simulink model "unifiedModle_IR_MAYBE"  (R2023b)
settings: Solver=FixedStepAuto  StartTime=0.0  StopTime=inf  RelTol=1e-3  EnableMultiTasking=on
libraries: vexarmcortexlib x28, vexcommonlib x8, simulink x3
settings Model: Creator=carol  LastModifiedBy=carol
settings SolverCC: AutoInsertRateTranBlk=on
settings DataIOCC: LimitDataPoints=on  SignalLoggingSaveFormat=ModelDataLogs  ReturnWorkspaceOutputs=off
settings OptimizationCC: ExpressionDepthLimit=2147483647  LifeSpan=Inf  MaxStackSize=64  EfficientTunableParamExpr=on
settings DebuggingCC: MergeDetectMultiDrivingBlocksExec=none  InheritedTsInSrcMsg=none  FcnCallInpInsideContextMsg=warning  StateNameClashWarn=warning  SFUnexpectedBacktrackingDiag=warning  SFNoUnconditionalDefaultTransitionDiag=warning  SFExecutionAtInitializationDiag=none  ArithmeticOperatorsInVariantConditions=warning
settings HardwareCC: ProdBitPerPointer=32  ProdBitPerSizeT=32  ProdBitPerPtrDiffT=32  ProdLargestAtomicInteger=Long  ProdLargestAtomicFloat=Double  ProdIntDivRoundTo=Undefined  ProdWordSize=32  ProdHWDeviceType=ARM Compatible->ARM Cortex
settings ModelReferenceCC: EnableRefExpFcnMdlSchedulingChecks=on  PropagateSignalLabelsOutOfModel=off
settings SFSimCC: MATLABDynamicMemAlloc=off  CustomCodeUndefinedFunction=UseInterfaceOnly
settings RTWCC: Description=Embedded Coder  SystemTargetFile=ert.tlc  HardwareBoard=ARM Cortex-based VEX Microcontroller  TemplateMakefile=ert_default_tmf  Toolchain=GNU Tools for VEX ARM Cortex
settings CodeAppCC: IgnoreCustomStorageClasses=off  CustomSymbolStrType=$N$R$M  StateflowObjectComments=on  InternalIdentifier=Classic
settings ERTTargetCC: CodeReplacementLibrary=GCC ARM Cortex-M3  MultiwordLength=2048  ConvertIfToSwitch=off  SuppressUnreachableDefaultCases=off

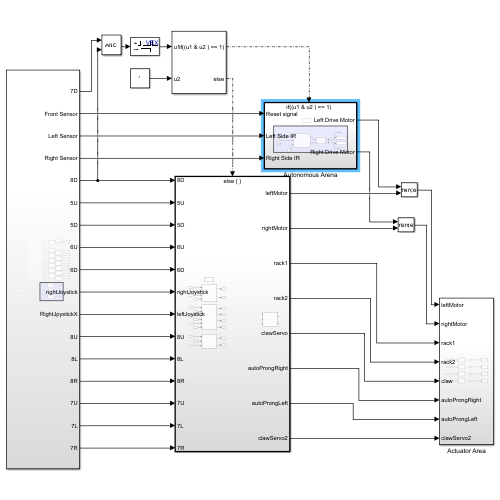
[thumbnail: Simulink's stored preview of the top-level diagram]
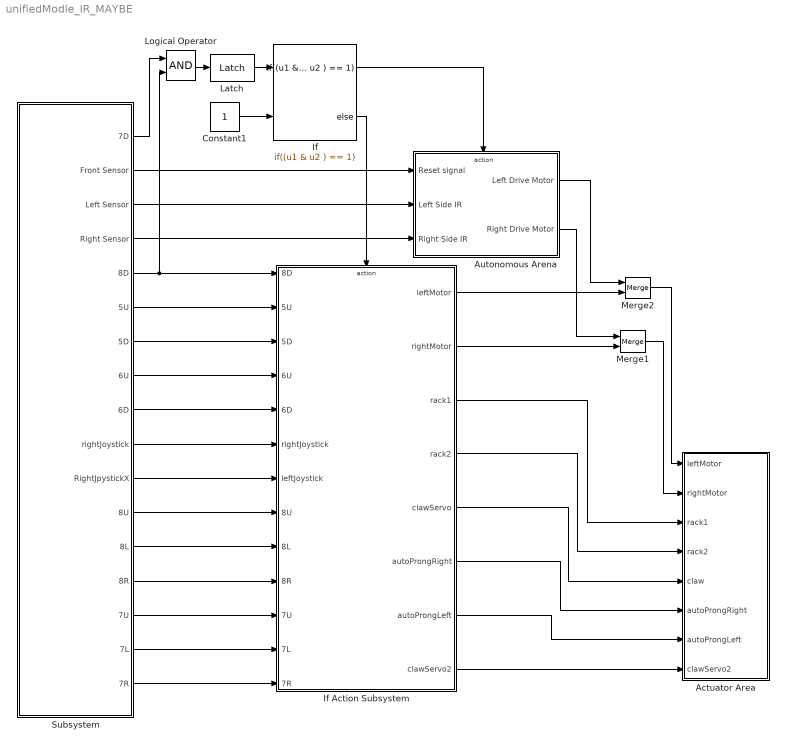
== system unifiedModle_IR_MAYBE ==
  Actuator Area : Subsystem
  Autonomous Arena : Subsystem  TreatAsAtomicUnit=on
  Constant1 : Constant
  If : If  NumInputs=2  IfExpression=(u1 & u2 ) == 1
  If Action Subsystem : Subsystem  TreatAsAtomicUnit=on
  Latch : vexcommonlib/Latch  output0=off  BlockPlatform=vexarmcortex
      settings: LibrarySourceBlock=vexarmcortexlib/Utilities/Latch
  Logical Operator : Logic  AllPortsSameDT=off  OutDataTypeStr=boolean
  Merge1 : Merge
  Merge2 : Merge
  Subsystem : Subsystem
  wires:
  If Action Subsystem/8(clawServo2) -> Actuator Area/8(clawServo2)
  If Action Subsystem/5(clawServo) -> Actuator Area/5(claw)
  If Action Subsystem/3(rack1) -> Actuator Area/3(rack1)
  If Action Subsystem/6(autoProngRight) -> Actuator Area/6(autoProngRight)
  If Action Subsystem/4(rack2) -> Actuator Area/4(rack2)
  If Action Subsystem/7(autoProngLeft) -> Actuator Area/7(autoProngLeft)
  If Action Subsystem/1(leftMotor) -> Merge2/2
  If Action Subsystem/2(rightMotor) -> Merge1/2
  Subsystem/5(8D) -> If Action Subsystem/1(8D), Logical Operator/2
  Subsystem/6(5U) -> If Action Subsystem/2(5U)
  Subsystem/7(5D) -> If Action Subsystem/3(5D)
  Subsystem/8(6U) -> If Action Subsystem/4(6U)
  Subsystem/9(6D) -> If Action Subsystem/5(6D)
  Subsystem/10(rightJoystick) -> If Action Subsystem/6(rightJoystick)
  Subsystem/11(RightJpystickX) -> If Action Subsystem/7(leftJoystick)
  Subsystem/12(8U) -> If Action Subsystem/8(8U)
  Subsystem/13(8L) -> If Action Subsystem/9(8L)
  Subsystem/14(8R) -> If Action Subsystem/10(8R)
  Subsystem/15(7U) -> If Action Subsystem/11(7U)
  Subsystem/16(7L) -> If Action Subsystem/12(7L)
  Subsystem/17(7R) -> If Action Subsystem/13(7R)
  Logical Operator/1 -> Latch/1
  Subsystem/1(7D) -> Logical Operator/1
  Latch/1 -> If/1
  Constant1/1 -> If/2
  Merge1/1 -> Actuator Area/2(rightMotor)
  Merge2/1 -> Actuator Area/1(leftMotor)
  Autonomous Arena/1(Left Drive Motor) -> Merge2/1
  Autonomous Arena/2(Right Drive Motor) -> Merge1/1
  Subsystem/4(Right Sensor) -> Autonomous Arena/3(Right Side IR)
  Subsystem/2(Front Sensor) -> Autonomous Arena/1(Reset signal)
  Subsystem/3(Left Sensor) -> Autonomous Arena/2(Left Side IR)
  If/1 -> Autonomous Arena/Action
  If/2 -> If Action Subsystem/Action

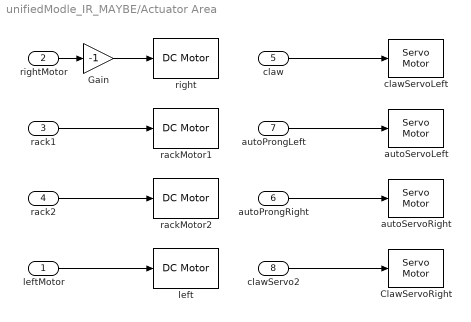
== system unifiedModle_IR_MAYBE/Actuator Area ==
  leftMotor : Inport
  rightMotor : Inport  Port=2
  rack1 : Inport  Port=3
  rack2 : Inport  Port=4
  claw : Inport  Port=5
  autoProngRight : Inport  Port=6
  autoProngLeft : Inport  Port=7
  clawServo2 : Inport  Port=8
  ClawServoRight : vexarmcortexlib/Actuators/Servo Motor  motor=8  scaleFactor=60/127  SimulationOut=off
  Gain : Gain  Gain=-1
  autoServoLeft : vexarmcortexlib/Actuators/Servo Motor  motor=4  scaleFactor=60/127  SimulationOut=off
  autoServoRight : vexarmcortexlib/Actuators/Servo Motor  motor=7  scaleFactor=60/127  SimulationOut=off
  clawServoLeft : vexarmcortexlib/Actuators/Servo Motor  motor=3  scaleFactor=60/127  SimulationOut=off
  left : vexarmcortexlib/Actuators/DC Motor  motor=9  scaleFactor=1/13.5  SimulationOut=off
  rackMotor1 : vexarmcortexlib/Actuators/DC Motor  motor=6  scaleFactor=1/13.5  SimulationOut=off
  rackMotor2 : vexarmcortexlib/Actuators/DC Motor  motor=5  scaleFactor=1/13.5  SimulationOut=off
  right : vexarmcortexlib/Actuators/DC Motor  motor=2  scaleFactor=1/13.5  SimulationOut=off
  wires:
  leftMotor/1 -> left/1
  autoProngLeft/1 -> autoServoLeft/1
  rack1/1 -> rackMotor1/1
  rightMotor/1 -> Gain/1
  autoProngRight/1 -> autoServoRight/1
  clawServo2/1 -> ClawServoRight/1
  claw/1 -> clawServoLeft/1
  rack2/1 -> rackMotor2/1
  Gain/1 -> right/1

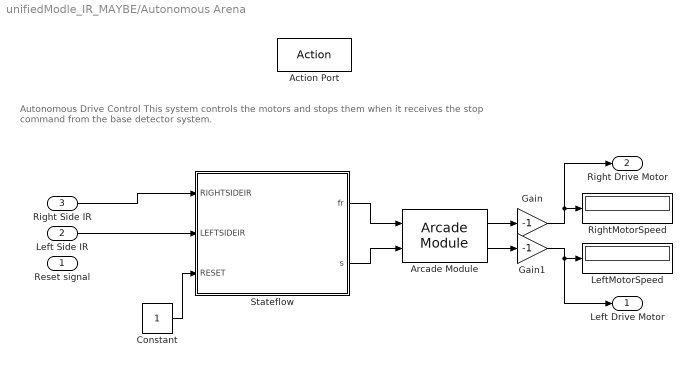
== system unifiedModle_IR_MAYBE/Autonomous Arena ==
  note: Autonomous Drive Control
      | This system controls the motors and stops them when it receives the stop command from the base detector system.
  Reset signal : Inport
  Left Side IR : Inport  Port=2
  Right Side IR : Inport  Port=3
  Action Port : ActionPort  ActionPortLabel=if((u1 & u2 ) == 1)
  Arcade Module : vexcommonlib/Arcade Module  BlockPlatform=vexarmcortex
  Constant : Constant
  Gain : Gain  Gain=-1
  Gain1 : Gain  Gain=-1
  LeftMotorSpeed : Display
  RightMotorSpeed : Display
  Stateflow : Stateflow chart  TreatAsAtomicUnit=on
  Left Drive Motor : Outport
  Right Drive Motor : Outport  Port=2
  wires:
  Arcade Module/1 -> Gain/1
  Stateflow/2(s) -> Arcade Module/2
  Stateflow/1(fr) -> Arcade Module/1
  Constant/1 -> Stateflow/3(RESET)
  Arcade Module/2 -> Gain1/1
  Gain1/1 -> LeftMotorSpeed/1, Left Drive Motor/1
  Gain/1 -> Right Drive Motor/1, RightMotorSpeed/1
  Right Side IR/1 -> Stateflow/1(RIGHTSIDEIR)
  Left Side IR/1 -> Stateflow/2(LEFTSIDEIR)

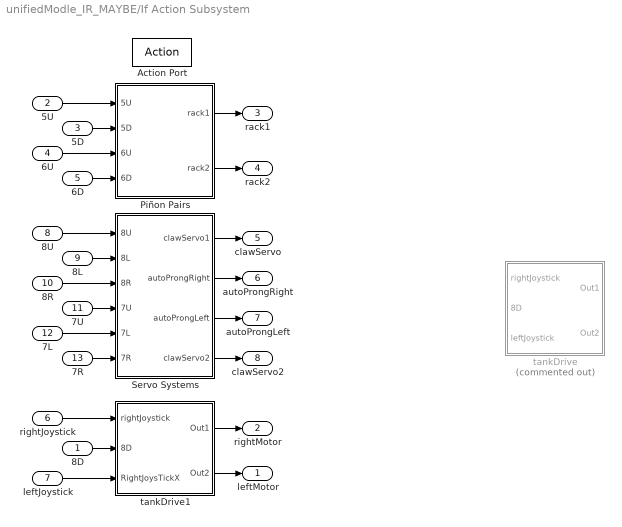
== system unifiedModle_IR_MAYBE/If Action Subsystem ==
  8D : Inport
  5U : Inport  Port=2
  5D : Inport  Port=3
  6U : Inport  Port=4
  6D : Inport  Port=5
  rightJoystick : Inport  Port=6
  leftJoystick : Inport  Port=7
  8U : Inport  Port=8
  8L : Inport  Port=9
  8R : Inport  Port=10
  7U : Inport  Port=11
  7L : Inport  Port=12
  7R : Inport  Port=13
  Action Port : ActionPort  ActionPortLabel=else
  Piñon Pairs : Subsystem
  Servo Systems : Subsystem
  tankDrive : Subsystem  Commented=on
  tankDrive1 : Subsystem
  leftMotor : Outport
  rightMotor : Outport  Port=2
  rack1 : Outport  Port=3
  rack2 : Outport  Port=4
  clawServo : Outport  Port=5
  autoProngRight : Outport  Port=6
  autoProngLeft : Outport  Port=7
  clawServo2 : Outport  Port=8
  wires:
  Servo Systems/2(autoProngRight) -> autoProngRight/1
  Servo Systems/4(clawServo2) -> clawServo2/1
  Servo Systems/3(autoProngLeft) -> autoProngLeft/1
  Servo Systems/1(clawServo1) -> clawServo/1
  7U/1 -> Servo Systems/4(7U)
  Piñon Pairs/1(rack1) -> rack1/1
  8U/1 -> Servo Systems/1(8U)
  7R/1 -> Servo Systems/6(7R)
  6U/1 -> Piñon Pairs/3(6U)
  Piñon Pairs/2(rack2) -> rack2/1
  6D/1 -> Piñon Pairs/4(6D)
  7L/1 -> Servo Systems/5(7L)
  5U/1 -> Piñon Pairs/1(5U)
  8R/1 -> Servo Systems/3(8R)
  5D/1 -> Piñon Pairs/2(5D)
  8L/1 -> Servo Systems/2(8L)
  8D/1 -> tankDrive1/2("8D ")
  tankDrive1/1(Out1) -> rightMotor/1
  tankDrive1/2(Out2) -> leftMotor/1
  rightJoystick/1 -> tankDrive1/1(rightJoystick)
  leftJoystick/1 -> tankDrive1/3(RightJoysTickX)

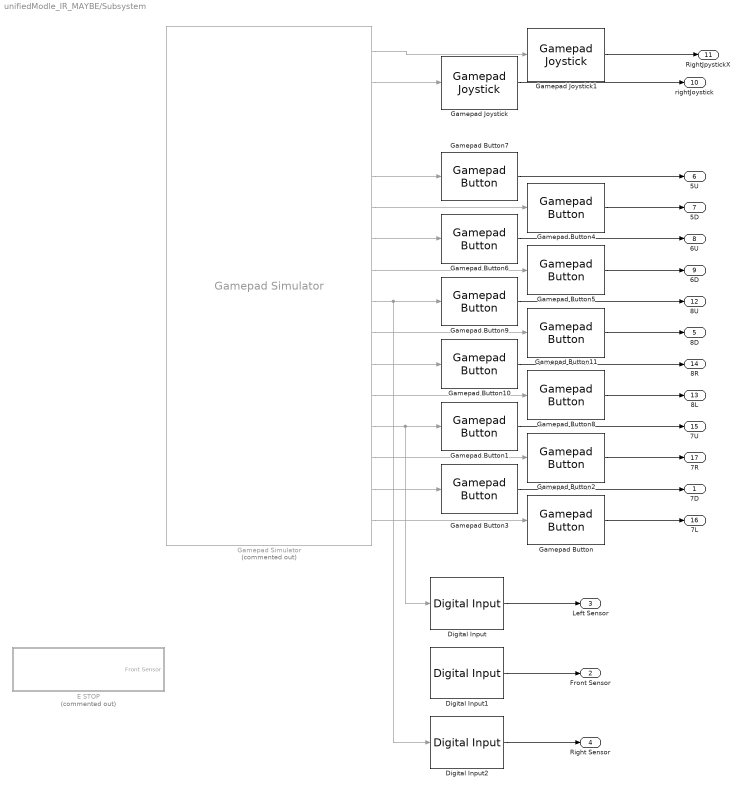
== system unifiedModle_IR_MAYBE/Subsystem ==
  Digital Input : vexarmcortexlib/Sensors/Digital Input  inChan=2  SimulationIn=on  SampleTime=.02
  Digital Input1 : vexarmcortexlib/Sensors/Digital Input  inChan=6  SimulationIn=off  SampleTime=0.2
  Digital Input2 : vexarmcortexlib/Sensors/Digital Input  inChan=11  SimulationIn=on  SampleTime=.02
  E STOP : Subsystem  Commented=on
  Gamepad Button : vexarmcortexlib/Gamepad/Gamepad Button  joystick=1  chan=7  button56=Up  button78=Left  SimulationIn=on  SampleTime=0.02
  Gamepad Button1 : vexarmcortexlib/Gamepad/Gamepad Button  joystick=1  chan=7  button56=Up  button78=Up  SimulationIn=on  SampleTime=0.02
  Gamepad Button10 : vexarmcortexlib/Gamepad/Gamepad Button  joystick=1  chan=8  button56=Up  button78=Right  SimulationIn=on  SampleTime=0.02
  Gamepad Button11 : vexarmcortexlib/Gamepad/Gamepad Button  joystick=1  chan=8  button56=Up  button78=Down  SimulationIn=on  SampleTime=0.02
  Gamepad Button2 : vexarmcortexlib/Gamepad/Gamepad Button  joystick=1  chan=7  button56=Up  button78=Right  SimulationIn=on  SampleTime=0.02
  Gamepad Button3 : vexarmcortexlib/Gamepad/Gamepad Button  joystick=1  chan=7  button56=Up  button78=Down  SimulationIn=on  SampleTime=0.02
  Gamepad Button4 : vexarmcortexlib/Gamepad/Gamepad Button  joystick=1  chan=5  button56=Down  button78=Down  SimulationIn=on  SampleTime=0.02
  Gamepad Button5 : vexarmcortexlib/Gamepad/Gamepad Button  joystick=1  chan=6  button56=Down  button78=Down  SimulationIn=on  SampleTime=0.02
  Gamepad Button6 : vexarmcortexlib/Gamepad/Gamepad Button  joystick=1  chan=6  button56=Up  button78=Down  SimulationIn=on  SampleTime=0.02
  Gamepad Button7 : vexarmcortexlib/Gamepad/Gamepad Button  joystick=1  chan=5  button56=Up  button78=Down  SimulationIn=on  SampleTime=0.02
  Gamepad Button8 : vexarmcortexlib/Gamepad/Gamepad Button  joystick=1  chan=8  button56=Up  button78=Left  SimulationIn=on  SampleTime=0.02
  Gamepad Button9 : vexarmcortexlib/Gamepad/Gamepad Button  joystick=1  chan=8  button56=Up  button78=Up  SimulationIn=on  SampleTime=0.02
  Gamepad Joystick : vexarmcortexlib/Gamepad/Gamepad Joystick  joystick=1  chan=2  SimulationIn=on  SampleTime=0.02
  Gamepad Joystick1 : vexarmcortexlib/Gamepad/Gamepad Joystick  joystick=1  chan=1  SimulationIn=on  SampleTime=0.02
  Gamepad Simulator : vexcommonlib/Gamepad Simulator  Commented=on  WhichPad=XBox Gamepad  JoyId=1  BlockPlatform=vexarmcortex
      settings: LibrarySourceBlock=vexarmcortexlib/Utilities/Gamepad Simulator
  7D : Outport
  Front Sensor : Outport  Port=2
  Left Sensor : Outport  Port=3
  Right Sensor : Outport  Port=4
  8D : Outport  Port=5
  5U : Outport  Port=6
  5D : Outport  Port=7
  6U : Outport  Port=8
  6D : Outport  Port=9
  rightJoystick : Outport  Port=10
  RightJpystickX : Outport  Port=11
  8U : Outport  Port=12
  8L : Outport  Port=13
  8R : Outport  Port=14
  7U : Outport  Port=15
  7L : Outport  Port=16
  7R : Outport  Port=17
  wires:
  Gamepad Joystick1/1 -> RightJpystickX/1
  Gamepad Simulator/12 -> Gamepad Button8/1
  Gamepad Simulator/8 -> Gamepad Button5/1
  Gamepad Joystick/1 -> rightJoystick/1
  Gamepad Simulator/7 -> Gamepad Button6/1
  Gamepad Button9/1 -> 8U/1
  Gamepad Button7/1 -> 5U/1
  Gamepad Button10/1 -> 8R/1
  Gamepad Button2/1 -> 7R/1
  Gamepad Simulator/11 -> Gamepad Button10/1
  Gamepad Simulator/14 -> Gamepad Button2/1
  Gamepad Button6/1 -> 6U/1
  Gamepad Button1/1 -> 7U/1
  Gamepad Simulator/5 -> Gamepad Button7/1
  Gamepad Button8/1 -> 8L/1
  Gamepad Simulator/2 -> Gamepad Joystick/1
  Gamepad Button11/1 -> 8D/1
  Gamepad Button/1 -> 7L/1
  Gamepad Button5/1 -> 6D/1
  Gamepad Simulator/13 -> Digital Input/1, Gamepad Button1/1
  Gamepad Button3/1 -> 7D/1
  Gamepad Button4/1 -> 5D/1
  Gamepad Simulator/6 -> Gamepad Button4/1
  Gamepad Simulator/9 -> Digital Input2/1, Gamepad Button9/1
  Gamepad Simulator/16 -> Gamepad Button/1
  Digital Input/1 -> Left Sensor/1
  Digital Input2/1 -> Right Sensor/1
  Digital Input1/1 -> Front Sensor/1
  Gamepad Simulator/10 -> Gamepad Button11/1
  Gamepad Simulator/15 -> Gamepad Button3/1
  Gamepad Simulator/1 -> Gamepad Joystick1/1

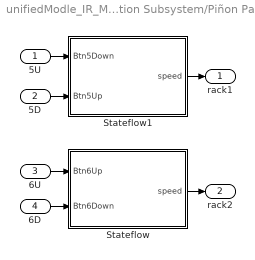
== system unifiedModle_IR_MAYBE/If Action Subsystem/Piñon Pairs ==
  5U : Inport
  5D : Inport  Port=2
  6U : Inport  Port=3
  6D : Inport  Port=4
  Stateflow : Stateflow chart  TreatAsAtomicUnit=on
  Stateflow1 : Stateflow chart  TreatAsAtomicUnit=on
  rack1 : Outport
  rack2 : Outport  Port=2
  wires:
  6U/1 -> Stateflow/1(Btn6Up)
  6D/1 -> Stateflow/2(Btn6Down)
  Stateflow/1(speed) -> rack2/1
  Stateflow1/1(speed) -> rack1/1
  5U/1 -> Stateflow1/1(Btn5Down)
  5D/1 -> Stateflow1/2(Btn5Up)

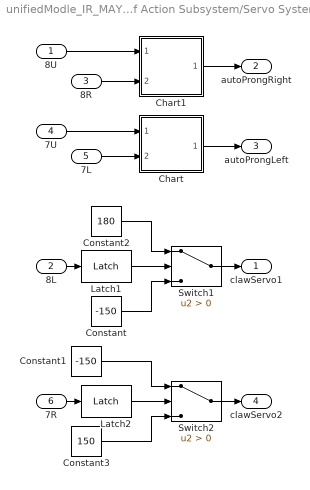
== system unifiedModle_IR_MAYBE/If Action Subsystem/Servo Systems ==
  8U : Inport
  8L : Inport  Port=2
  8R : Inport  Port=3
  7U : Inport  Port=4
  7L : Inport  Port=5
  7R : Inport  Port=6
  Chart : Stateflow chart  TreatAsAtomicUnit=on
  Chart1 : Stateflow chart  TreatAsAtomicUnit=on
  Constant : Constant  Value=-150
  Constant1 : Constant  Value=-150
  Constant2 : Constant  Value=180
  Constant3 : Constant  Value=150
  Latch1 : vexcommonlib/Latch  output0=off  BlockPlatform=vexarmcortex
      settings: LibrarySourceBlock=vexarmcortexlib/Utilities/Latch
  Latch2 : vexcommonlib/Latch  output0=off  BlockPlatform=vexarmcortex
      settings: LibrarySourceBlock=vexarmcortexlib/Utilities/Latch
  Switch1 : Switch  Criteria=u2 > Threshold  SaturateOnIntegerOverflow=off  InputSameDT=off
  Switch2 : Switch  Criteria=u2 > Threshold  SaturateOnIntegerOverflow=off  InputSameDT=off
  clawServo1 : Outport
  autoProngRight : Outport  Port=2
  autoProngLeft : Outport  Port=3
  clawServo2 : Outport  Port=4
  wires:
  Switch1/1 -> clawServo1/1
  8L/1 -> Latch1/1
  Constant2/1 -> Switch1/1
  Constant/1 -> Switch1/3
  Chart/1(angle) -> autoProngLeft/1
  7L/1 -> Chart/2(Btn7Left)
  7U/1 -> Chart/1(Btn7Up)
  Chart1/1(angle) -> autoProngRight/1
  8R/1 -> Chart1/2(Btn8Right)
  8U/1 -> Chart1/1(Btn8Up)
  Latch1/1 -> Switch1/2
  Latch2/1 -> Switch2/2
  Constant1/1 -> Switch2/1
  Constant3/1 -> Switch2/3
  Switch2/1 -> clawServo2/1
  7R/1 -> Latch2/1

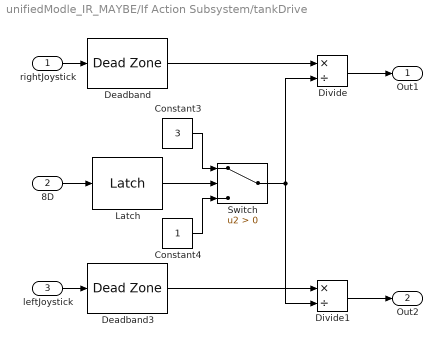
== system unifiedModle_IR_MAYBE/If Action Subsystem/tankDrive ==
  rightJoystick : Inport
  "8D " : Inport  Port=2
  leftJoystick : Inport  Port=3
  Constant3 : Constant  Value=3
  Constant4 : Constant
  Deadband : DeadZone  LowerValue=-9  UpperValue=9
  Deadband3 : DeadZone  LowerValue=-9  UpperValue=9
  Divide : Product  Inputs=*/
  Divide1 : Product  Inputs=*/
  Latch : vexcommonlib/Latch  output0=off  BlockPlatform=vexarmcortex
      settings: LibrarySourceBlock=vexarmcortexlib/Utilities/Latch
  Switch : Switch  Criteria=u2 > Threshold  SaturateOnIntegerOverflow=off  InputSameDT=off
  Out1 : Outport
  Out2 : Outport  Port=2
  wires:
  Constant4/1 -> Switch/3
  Constant3/1 -> Switch/1
  Divide1/1 -> Out2/1
  Latch/1 -> Switch/2
  Deadband3/1 -> Divide1/1
  Deadband/1 -> Divide/1
  Switch/1 -> Divide1/2, Divide/2
  rightJoystick/1 -> Deadband/1
  Divide/1 -> Out1/1
  "8D "/1 -> Latch/1
  leftJoystick/1 -> Deadband3/1

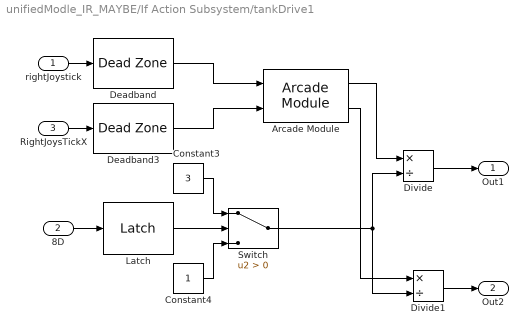
== system unifiedModle_IR_MAYBE/If Action Subsystem/tankDrive1 ==
  rightJoystick : Inport
  "8D " : Inport  Port=2
  RightJoysTickX : Inport  Port=3
  Arcade Module : vexcommonlib/Arcade Module  BlockPlatform=vexarmcortex
  Constant3 : Constant  Value=3
  Constant4 : Constant
  Deadband : DeadZone  LowerValue=-9  UpperValue=9
  Deadband3 : DeadZone  LowerValue=-9  UpperValue=9
  Divide : Product  Inputs=*/
  Divide1 : Product  Inputs=*/
  Latch : vexcommonlib/Latch  output0=off  BlockPlatform=vexarmcortex
      settings: LibrarySourceBlock=vexarmcortexlib/Utilities/Latch
  Switch : Switch  Criteria=u2 > Threshold  SaturateOnIntegerOverflow=off  InputSameDT=off
  Out1 : Outport
  Out2 : Outport  Port=2
  wires:
  Constant4/1 -> Switch/3
  Constant3/1 -> Switch/1
  Latch/1 -> Switch/2
  Deadband/1 -> Arcade Module/1
  rightJoystick/1 -> Deadband/1
  Divide/1 -> Out1/1
  "8D "/1 -> Latch/1
  RightJoysTickX/1 -> Deadband3/1
  Divide1/1 -> Out2/1
  Arcade Module/2 -> Divide1/1
  Arcade Module/1 -> Divide/1
  Deadband3/1 -> Arcade Module/2
  Switch/1 -> Divide/2, Divide1/2

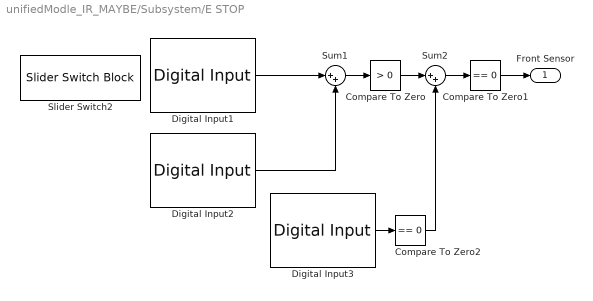
== system unifiedModle_IR_MAYBE/Subsystem/E STOP ==
  Compare To Zero : simulink/Logic and Bit Operations/Compare To Zero  relop=>  OutDataTypeStr=uint8
  Compare To Zero1 : simulink/Logic and Bit Operations/Compare To Zero  relop===  OutDataTypeStr=uint8
  Compare To Zero2 : simulink/Logic and Bit Operations/Compare To Zero  relop===  OutDataTypeStr=uint8
  Digital Input1 : vexarmcortexlib/Sensors/Digital Input  inChan=5  SimulationIn=off  SampleTime=0.2
  Digital Input2 : vexarmcortexlib/Sensors/Digital Input  inChan=6  SimulationIn=off  SampleTime=0.2
  Digital Input3 : vexarmcortexlib/Sensors/Digital Input  inChan=7  SimulationIn=off  SampleTime=0.2
  Slider Switch2 : SliderSwitchBlock
      settings: Values={{'Off', 'On'}, [0 1]}
  Sum1 : Sum  Inputs=|++
  Sum2 : Sum  Inputs=|++
  Front Sensor : Outport
  wires:
  Digital Input1/1 -> Sum1/1
  Sum1/1 -> Compare To Zero/1
  Digital Input2/1 -> Sum1/2
  Compare To Zero/1 -> Sum2/1
  Sum2/1 -> Compare To Zero1/1
  Compare To Zero1/1 -> Front Sensor/1
  Digital Input3/1 -> Compare To Zero2/1
  Compare To Zero2/1 -> Sum2/2

== stateflow chart unifiedModle_IR_MAYBE/If Action Subsystem/Piñon Pairs/Stateflow1 ==
  state rackIN
    entry:
    speed=-127;
  state STOPPED
    entry:
    speed=0;
  state rackOUT
    entry:
    speed=127;
  (default) -> STOPPED
  STOPPED -> rackOUT [order 2] : [Btn5Down==0 && Btn5Up==1]
  STOPPED -> rackIN [order 1] : [Btn5Down==1 && Btn5Up==0]
  rackIN -> STOPPED [order 1] : [Btn5Down==0]
  rackOUT -> STOPPED [order 1] : [Btn5Up==0]
  rackIN -> STOPPED [order 2] : [Btn5Down==1 && Btn5Up==1]
  rackOUT -> STOPPED [order 2] : [Btn5Down==1 && Btn5Up==1]
  data: speed output; Btn5Down input; Btn5Up input

== stateflow chart unifiedModle_IR_MAYBE/Autonomous Arena/Stateflow ==
  state STRAIGHT
    entry:
    fr = 90;
    s = 0;
  state GO_RIGHT
    entry:
    fr = 110;
    s = -90;
  state GO_LEFT
    entry:
    fr = 110;
    s = 90;
  state STOP
    entry:
    fr = 0;
    s = 0;
  (default) -> STRAIGHT
  GO_LEFT -> STRAIGHT [order 3] : [LEFTSIDEIR == 0 && RIGHTSIDEIR == 0]
  GO_RIGHT -> STRAIGHT [order 3] : [RIGHTSIDEIR == 0 && LEFTSIDEIR == 0]
  STRAIGHT -> GO_RIGHT [order 3] : [RIGHTSIDEIR == 0 && LEFTSIDEIR == 1]
  STRAIGHT -> GO_LEFT [order 2] : [LEFTSIDEIR == 0 && RIGHTSIDEIR ==1]
  STOP -> STRAIGHT [order 3] : [RIGHTSIDEIR == 0 && LEFTSIDEIR == 0 && RESET == 1]
  STRAIGHT -> STOP [order 1] : [RESET == 0]
  GO_LEFT -> GO_RIGHT [order 2] : [LEFTSIDEIR == 1 && RIGHTSIDEIR == 0]
  GO_RIGHT -> GO_LEFT [order 2] : [RIGHTSIDEIR == 1 && LEFTSIDEIR == 0]
  STOP -> GO_LEFT [order 2] : [RESET == 1 && LEFTSIDEIR == 0]
  GO_LEFT -> STOP [order 1] : [RESET == 0]
  STOP -> GO_RIGHT [order 1] : [RESET == 1 && RIGHTSIDEIR == 0]
  GO_RIGHT -> STOP [order 1] : [RESET == 0]
  data: RIGHTSIDEIR input; LEFTSIDEIR input; RESET input; fr output; s output

== stateflow chart unifiedModle_IR_MAYBE/If Action Subsystem/Servo Systems/Chart1 ==
  state neutral
    angle=0;
  state buffer
    angle=0;
  state negative90
    angle=-30;
  state positive90
    angle=50;
  (default) -> neutral
  neutral -> negative90 [order 1] : [Btn8Right==1 && Btn8Up==0]
  neutral -> positive90 [order 2] : [Btn8Up==1 && Btn8Right==0]
  buffer -> neutral : [after(.75,sec)]
  positive90 -> buffer [order 1] : [Btn8Up==1 && Btn8Right==1]
  negative90 -> buffer [order 1] : [Btn8Right==1 && Btn8Up==1]
  negative90 -> positive90 [order 2] : [Btn8Right==0 && Btn8Up==1]
  positive90 -> negative90 [order 2] : [Btn8Up==0 && Btn8Right==1]
  data: angle output; Btn8Up input; Btn8Right input

== stateflow chart unifiedModle_IR_MAYBE/If Action Subsystem/Servo Systems/Chart ==
  state neutral
    angle=3;
  state buffer
    angle=3;
  state negative90
    angle=-40;
  state positive90
    angle=50;
  (default) -> neutral
  neutral -> negative90 [order 1] : [Btn7Left==1 && Btn7Up==0]
  neutral -> positive90 [order 2] : [Btn7Up==1 && Btn7Left==0]
  buffer -> neutral : [after(.75,sec)]
  negative90 -> buffer [order 1] : [Btn7Left==1 && Btn7Up==1]
  positive90 -> buffer [order 1] : [Btn7Up==1 && Btn7Left==1]
  negative90 -> positive90 [order 2] : [Btn7Left==0 && Btn7Up==1]
  positive90 -> negative90 [order 2] : [Btn7Up==0 && Btn7Left==1]
  data: Btn7Up input; Btn7Left input; angle output

== stateflow chart unifiedModle_IR_MAYBE/If Action Subsystem/Piñon Pairs/Stateflow ==
  state rackIN
    entry:
    speed=-127;
  state STOPPED
    entry:
    speed=20;
  state rackOUT
    entry:
    speed=127;
  (default) -> STOPPED
  STOPPED -> rackOUT [order 2] : [Btn6Down==0 && Btn6Up==1]
  STOPPED -> rackIN [order 1] : [Btn6Down==1 && Btn6Up==0]
  rackIN -> STOPPED [order 1] : [Btn6Down==0]
  rackOUT -> STOPPED [order 1] : [Btn6Up==0]
  rackIN -> STOPPED [order 2] : [Btn6Down==1 && Btn6Up==1]
  rackOUT -> STOPPED [order 2] : [Btn6Down==1 && Btn6Up==1]
  data: Btn6Up input; Btn6Down input; speed output
